simulink model "termin2v4_vorgabe"  (Simulink 7.0)
settings: Solver=FixedStepDiscrete  SolverMode=SingleTasking  StartTime=0.0  StopTime=512/8000  RelTol=1e-3  AbsTol=1e-6
undefined symbols (not defined in the file or in its folder): Fs, get
libraries: dspsnks4 x4, dspbuff3 x2, dspxfrm3 x2, dspsrcs4 x2
settings Model: Creator=dsv1_4  LastModifiedBy=dsv1_4  ExtModeTrigMode=oneshot  ExtModeArmWhenConnect=off
settings DataIOCC: LimitDataPoints=off  SignalLoggingName=sigsOut
settings OptimizationCC: BooleanDataType=off
settings DebuggingCC: SaveWithParameterizedLinksMsg=none  SignalResolutionControl=TryResolveAllWithWarning  SolverPrmCheckMsg=none  MultiTaskDSMMsg=warning  MultiTaskCondExecSysMsg=none  StrictBusMsg=None
settings HardwareCC: TargetUnknown=on
settings RTWCC: IncludeERTFirstTime=on
settings GRTTargetCC: TargetFcnLib=ansi_tfl_tmw.mat

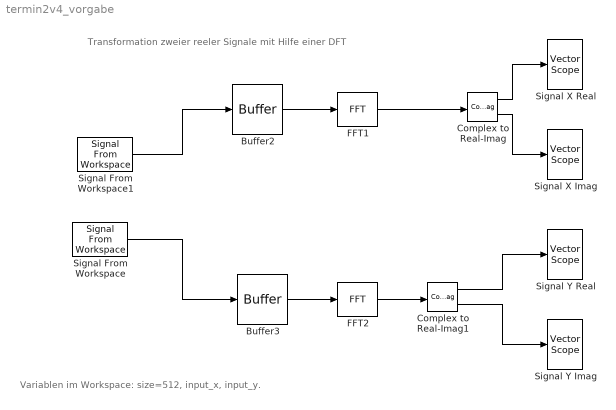
== system termin2v4_vorgabe ==
  note: Transformation zweier reeler Signale mit Hilfe einer DFT
  note: Variablen im Workspace:
      | size=512,
      | input_x,
      | input_y.
  Buffer2 : dspbuff3/Buffer  N=512  V=0  ic=0
  Buffer3 : dspbuff3/Buffer  N=512  V=0  ic=0
  Complex to Real-Imag : ComplexToRealImag
  Complex to Real-Imag1 : ComplexToRealImag
  FFT1 : dspxfrm3/FFT  DialogController=dspDDGCreate  DialogControllerArgs=DataTag0  CompMethod=Table lookup  TableOpt=Speed  BitRevOrder=off  InheritFFTLength=on  FFTLength=64  SkipNorm=on  roundingMode=Floor  overflowMode=off
  FFT2 : dspxfrm3/FFT  DialogController=dspDDGCreate  DialogControllerArgs=DataTag1  CompMethod=Table lookup  TableOpt=Speed  BitRevOrder=off  InheritFFTLength=on  FFTLength=64  SkipNorm=on  roundingMode=Floor  overflowMode=off
  Signal From Workspace : dspsrcs4/Signal From Workspace  SystemSampleTime=-1  X=input_y  Ts=1/8000  nsamps=1  OutputAfterFinalValue=Setting to zero  ignoreOrWarnInputAndFrameLengths=off
  Signal From Workspace1 : dspsrcs4/Signal From Workspace  SystemSampleTime=-1  X=input_x  Ts=1/8000  nsamps=1  OutputAfterFinalValue=Setting to zero  ignoreOrWarnInputAndFrameLengths=off
  Signal X Imag : dspsnks4/Vector Scope  DialogController=dspdialog.VectorScope  DialogControllerArgs=DataTag2  ScopeProperties=off  Domain=Frequency  HorizSpan=1  DisplayProperties=off  AxisGrid=on  Memory=off  FrameNumber=on  AxisLegend=off  AxisZoom=off  OpenScopeAtSimStart=on  OpenScopeImmediately=off  FigPos=get(0,'defaultfigureposition')  AxisProperties=on  XUnits=Hertz  XRange=[-Fs/2...Fs/2]  InheritXIncr=on  XIncr=1  XLabel=Time  XLimit=Auto  XMin=0  XMax=1  XStart=0  YUnits=Magnitude  YLabel=Amplitude  LineProperties=off
      settings: YMin=-10  YMax=10
  Signal X Real : dspsnks4/Vector Scope  DialogController=dspdialog.VectorScope  DialogControllerArgs=DataTag3  ScopeProperties=off  Domain=Frequency  HorizSpan=1  DisplayProperties=off  AxisGrid=on  Memory=off  FrameNumber=on  AxisLegend=off  AxisZoom=off  OpenScopeAtSimStart=on  OpenScopeImmediately=off  FigPos=get(0,'defaultfigureposition')  AxisProperties=on  XUnits=Hertz  XRange=[-Fs/2...Fs/2]  InheritXIncr=on  XIncr=1  XLabel=Time  XLimit=Auto  XMin=0  XMax=1  XStart=0  YUnits=Magnitude  YLabel=Amplitude  LineProperties=off
      settings: YMin=-10  YMax=10
  Signal Y Imag : dspsnks4/Vector Scope  DialogController=dspdialog.VectorScope  DialogControllerArgs=DataTag4  ScopeProperties=off  Domain=Frequency  HorizSpan=1  DisplayProperties=off  AxisGrid=on  Memory=off  FrameNumber=on  AxisLegend=off  AxisZoom=off  OpenScopeAtSimStart=on  OpenScopeImmediately=off  FigPos=get(0,'defaultfigureposition')  AxisProperties=on  XUnits=Hertz  XRange=[-Fs/2...Fs/2]  InheritXIncr=on  XIncr=1  XLabel=Time  XLimit=Auto  XMin=0  XMax=1  XStart=0  YUnits=Magnitude  YLabel=Amplitude  LineProperties=off
      settings: YMin=-10  YMax=10
  Signal Y Real : dspsnks4/Vector Scope  DialogController=dspdialog.VectorScope  DialogControllerArgs=DataTag5  ScopeProperties=off  Domain=Frequency  HorizSpan=1  DisplayProperties=off  AxisGrid=on  Memory=off  FrameNumber=on  AxisLegend=off  AxisZoom=off  OpenScopeAtSimStart=on  OpenScopeImmediately=off  FigPos=get(0,'defaultfigureposition')  AxisProperties=on  XUnits=Hertz  XRange=[-Fs/2...Fs/2]  InheritXIncr=on  XIncr=1  XLabel=Time  XLimit=Auto  XMin=0  XMax=1  XStart=0  YUnits=Magnitude  YLabel=Amplitude  LineProperties=off
      settings: YMin=-10  YMax=10
  wires:
  Buffer2/1 -> FFT1/1
  Buffer3/1 -> FFT2/1
  FFT1/1 -> Complex to Real-Imag/1
  FFT2/1 -> Complex to Real-Imag1/1
  Complex to Real-Imag/1 -> Signal X Real/1
  Complex to Real-Imag1/2 -> Signal Y Imag/1
  Signal From Workspace1/1 -> Buffer2/1
  Signal From Workspace/1 -> Buffer3/1
  Complex to Real-Imag/2 -> Signal X Imag/1
  Complex to Real-Imag1/1 -> Signal Y Real/1
